simulink model "TD2"  (Simulink 9.0)
settings: Solver=ode23t  StartTime=0.0  StopTime=1  RelTol=1e-3
InitFcn:
  | TD2_config
StartFcn:
  | TD2_config
values from neighbouring files (symbols this model uses):
  b = 3.5077E-6    (= 3.5077e-06)    [MCC_constants.m]    (also in TD2_config.m = 0.0085)
  J = 3.2248E-6    (= 3.2248e-06)    [MCC_constants.m]    (also in TD2_config.m = 0.28)
  K = 0.0274    [MCC_constants.m]    (also in TD2_config.m = 0.5093)
  Kd = 0.1    [TD2_config.m]
  KdPos = 0.2    [TD2_config.m]
  Ki = 25    [TD2_config.m]
  KiPos = 10    [TD2_config.m]
  Kp = 6    [TD2_config.m]
  KpPos = 50    [TD2_config.m]
  L = 2.75E-6    (= 2.75e-06)    [MCC_constants.m]    (also in TD2_config.m = 0.0016)
  R = 4    [MCC_constants.m]    (also in TD2_config.m = 0.02)
libraries: simulink x1
settings Model: Creator=GEII Robot  LastModifiedBy=GEII Robot
settings DataIOCC: SaveFormat=Dataset
settings OptimizationCC: LifeSpan=auto
settings DebuggingCC: UnderspecifiedInitializationDetection=Simplified  MergeDetectMultiDrivingBlocksExec=error  SFUnexpectedBacktrackingDiag=error  SFNoUnconditionalDefaultTransitionDiag=error  SFExecutionAtInitializationDiag=warning
settings HardwareCC: ProdBitPerPointer=64  ProdBitPerSizeT=64  ProdBitPerPtrDiffT=64  ProdLargestAtomicFloat=Float  ProdIntDivRoundTo=Zero  ProdEndianess=LittleEndian  ProdWordSize=64  ProdHWDeviceType=Intel->x86-64 (Windows64)
settings ModelReferenceCC: PropagateSignalLabelsOutOfModel=on
settings CodeAppCC: StateflowObjectComments=off
settings GRTTargetCC: TargetLangStandard=C99 (ISO)
settings ConfigComp: CovMetricSettings=dwe  CovHtmlReporting=off  CovSaveCumulativeToWorkspaceVar=off  CovSaveSingleToWorkspaceVar=off  CovExternalEMLEnable=on

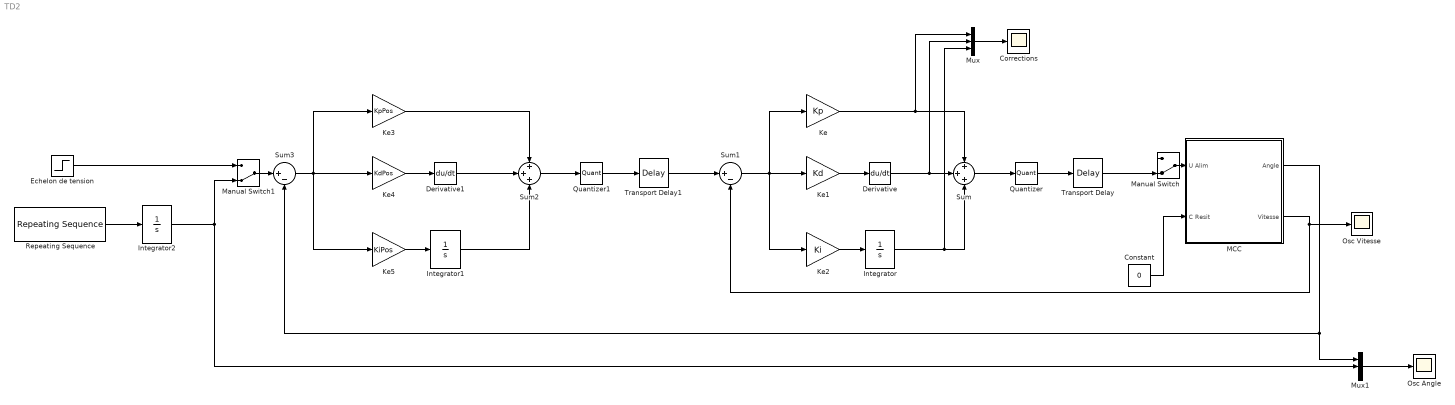
== system TD2 ==
  Constant : Constant  Value=0
  Corrections : Scope
  Derivative : Derivative
  Derivative1 : Derivative
  Echelon de tension : Step  Time=0  SampleTime=0
  Integrator : Integrator
  Integrator1 : Integrator
  Integrator2 : Integrator
  Ke : Gain  Gain=Kp
  Ke1 : Gain  Gain=Kd
  Ke2 : Gain  Gain=Ki
  Ke3 : Gain  Gain=KpPos
  Ke4 : Gain  Gain=KdPos
  Ke5 : Gain  Gain=KiPos
  MCC : Subsystem
  Manual Switch : ManualSwitch  CurrentSetting=0
  Manual Switch1 : ManualSwitch  CurrentSetting=0
  Mux : Mux  Inputs=3
  Mux1 : Mux  Inputs=3
  Osc Angle : Scope
  Osc Vitesse : Scope
  Quantizer : Quantizer  QuantizationInterval=0.004
  Quantizer1 : Quantizer  QuantizationInterval=0.05
  Repeating Sequence : simulink/Sources/Repeating Sequence  rep_seq_t=[0 0.1 0.2 0.3 0.8]  rep_seq_y=[0 5 5 0 0]
  Sum : Sum  Inputs=+++
  Sum1 : Sum  Inputs=|+-
  Sum2 : Sum  Inputs=+++
  Sum3 : Sum  Inputs=|+-
  Transport Delay : TransportDelay  DelayTime=0.001
  Transport Delay1 : TransportDelay  DelayTime=0.02
  wires:
  MCC/2(Vitesse) -> Osc Vitesse/1, Sum1/2
  Ke2/1 -> Integrator/1
  Integrator/1 -> Mux/3, Sum/3
  Ke/1 -> Mux/1, Sum/1
  Ke1/1 -> Derivative/1
  Derivative/1 -> Mux/2, Sum/2
  Constant/1 -> MCC/2(C Resit)
  Sum1/1 -> Ke/1, Ke2/1, Ke1/1
  Mux/1 -> Corrections/1
  Manual Switch/1 -> MCC/1(U Alim)
  Sum/1 -> Quantizer/1
  Quantizer/1 -> Transport Delay/1
  Transport Delay/1 -> Manual Switch/2
  Echelon de tension/1 -> Manual Switch1/1
  Repeating Sequence/1 -> Integrator2/1
  MCC/1(Angle) -> Sum3/2, Mux1/1
  Ke5/1 -> Integrator1/1
  Ke3/1 -> Sum2/1
  Derivative1/1 -> Sum2/2
  Integrator1/1 -> Sum2/3
  Ke4/1 -> Derivative1/1
  Sum2/1 -> Quantizer1/1
  Quantizer1/1 -> Transport Delay1/1
  Transport Delay1/1 -> Sum1/1
  Integrator2/1 -> Mux1/2, Manual Switch1/2
  Mux1/1 -> Osc Angle/1
  Manual Switch1/1 -> Sum3/1
  Sum3/1 -> Ke5/1, Ke3/1, Ke4/1

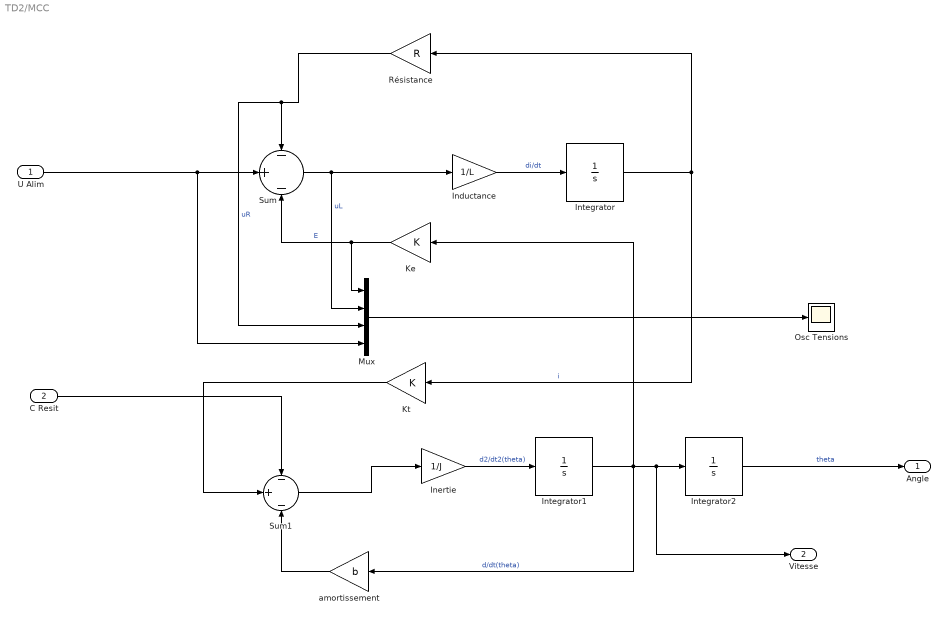
== system TD2/MCC ==
  U Alim : Inport
  C Resit : Inport  Port=2
  Inductance : Gain  Gain=1/L
  Inertie : Gain  Gain=1/J
  Integrator : Integrator
  Integrator1 : Integrator
  Integrator2 : Integrator
  Ke : Gain  Gain=K
  Kt : Gain  Gain=K
  Mux : Mux
  Osc Tensions : Scope
  Résistance : Gain  Gain=R
  Sum : Sum  Inputs=-|+|-
  Sum1 : Sum  Inputs=-|+|-
  amortissement : Gain  Gain=b
  Angle : Outport
  Vitesse : Outport  Port=2
  wires:
  Mux/1 -> Osc Tensions/1
  Sum1/1 -> Inertie/1
  Inertie/1 -> Integrator1/1  "d2/dt2(theta)"
  Integrator2/1 -> Angle/1  "theta"
  C Resit/1 -> Sum1/1
  amortissement/1 -> Sum1/3
  Ke/1 -> Mux/1, Sum/3  "E"
  U Alim/1 -> Mux/4, Sum/2
  Kt/1 -> Sum1/2
  Résistance/1 -> Mux/3, Sum/1  "uR"
  Integrator/1 -> Résistance/1, Kt/1  "i"
  Integrator1/1 -> amortissement/1, Ke/1, Vitesse/1, Integrator2/1  "d/dt(theta)"
  Sum/1 -> Inductance/1, Mux/2  "uL"
  Inductance/1 -> Integrator/1  "di/dt"
